simulink model "final_part_5"  (Simulink 8.3)
settings: Solver=ode45  StartTime=0.0  StopTime=60  RelTol=1e-3
undefined symbols (not defined in the file or in its folder): ctrl_est, drawMass, P
settings Model: Creator=beard  LastModifiedBy=jhl48
settings DataIOCC: LimitDataPoints=off
settings OptimizationCC: ExpressionDepthLimit=2147483647
settings DebuggingCC: SolverPrmCheckMsg=none  FcnCallInpInsideContextMsg=UseLocalSettings

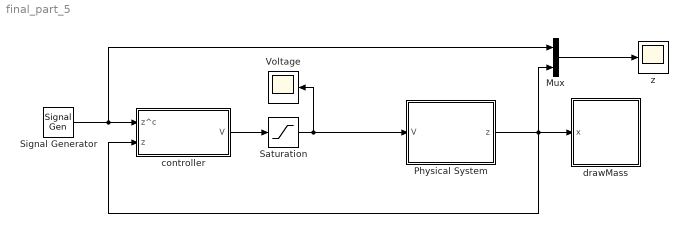
== system final_part_5 ==
  Mux : Mux  Inputs=2
  Physical System : Subsystem
  Saturation : Saturate  UpperLimit=P.V_max  LowerLimit=-P.V_max
  Signal Generator : SignalGenerator  WaveForm=square  Amplitude=0.5  Frequency=.025
  Voltage : Scope
      settings: TimeRange=60  YMin=-4  YMax=-3  SaveName=ScopeData2
  controller : Subsystem
  drawMass : Subsystem
      mask init:
      | % drawing parameters
      | L = 5;
      | w = 1;
      | theta = 45*pi/180;
      mask Display: image(imread('tv.jpg'))
  z : Scope
      settings: TimeRange=60  YMin=-0.75  YMax=0.75
  wires:
  Mux/1 -> z/1
  controller/1(V) -> Saturation/1
  Signal Generator/1 -> controller/1(z^c), Mux/1
  Physical System/1(z) -> controller/2(z), Mux/2, drawMass/1(x)
  Saturation/1 -> Physical System/1(V), Voltage/1

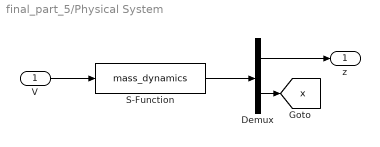
== system final_part_5/Physical System ==
  V : Inport
  Demux : Demux  Outputs=[1;3]
  S-Function : S-Function  FunctionName=mass_dynamics  Parameters=P  EnableBusSupport=off
  z : Outport
  tag scope: x=global
  wires:
  Demux/1 -> z/1
  Demux/2 -> [x]
  S-Function/1 -> Demux/1
  V/1 -> S-Function/1

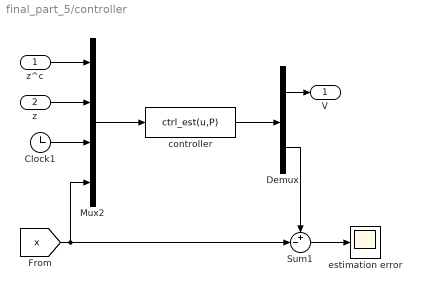
== system final_part_5/controller ==
  z^c : Inport
  z : Inport  Port=2
  Clock1 : Clock
  Demux : Demux  Outputs=[1;3]
  Mux2 : Mux
  Sum1 : Sum  Inputs=+-|
  controller : MATLABFcn  MATLABFcn=ctrl_est(u,P)  OutputDimensions=4  SampleTime=P.Ts
  estimation error : Scope
      settings: TimeRange=60  YMin=-0.004  YMax=0.004
  V : Outport
  wires:
  Mux2/1 -> controller/1
  z^c/1 -> Mux2/1
  z/1 -> Mux2/2
  Clock1/1 -> Mux2/3
  controller/1 -> Demux/1
  Demux/1 -> V/1
  Demux/2 -> Sum1/1
  Sum1/1 -> estimation error/1
  [x] -> Mux2/4, Sum1/2

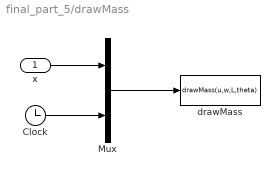
== system final_part_5/drawMass ==
  x : Inport
  Clock : Clock
  Mux : Mux  Inputs=2
  drawMass : MATLABFcn  MATLABFcn=drawMass(u,w,L,theta)  OutputDimensions=0  SampleTime=0.1
  wires:
  Mux/1 -> drawMass/1
  x/1 -> Mux/1
  Clock/1 -> Mux/2
